simulink model "test_path_detector"  (Simulink 7.6)
settings: Solver=FixedStepDiscrete  StartTime=0.0  StopTime=0  RelTol=1e-3
undefined symbols (not defined in the file or in its folder): gray, Rec, Scale_Down_B, Scale_Down_G, Scale_Down_H, Scale_Down_R, Scale_Down_S, Scale_Down_V, SDTV
libraries: vipsnks x12, vipconversions x2, vipsrcs x1, viptextngfix x1
settings Model: Creator=Thing 1  LastModifiedBy=auvt
settings RTWCC: TargetLang=C++

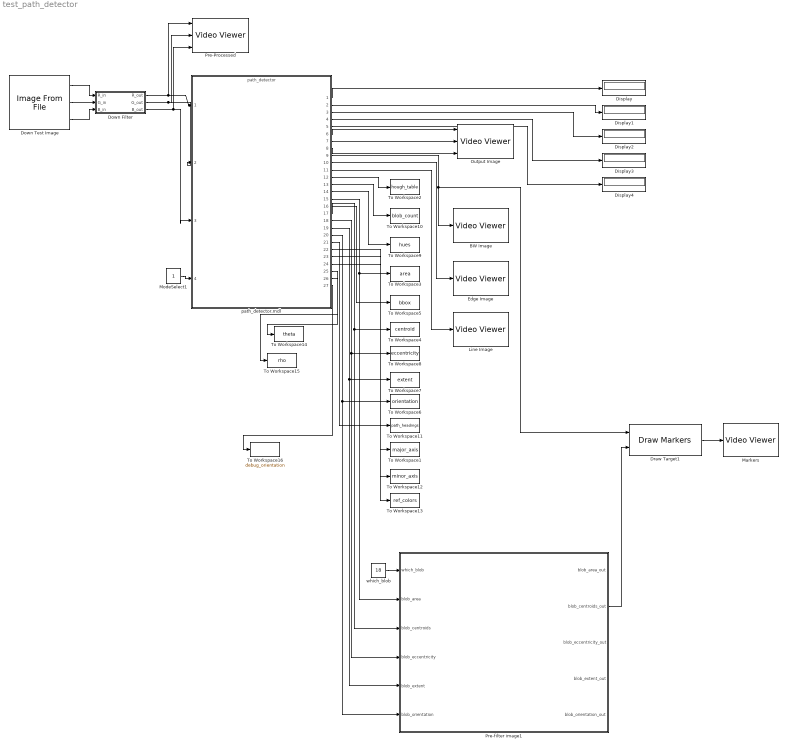
== system test_path_detector ==
  BW Image : vipsnks/Video Viewer  DialogControllerArgs=DataTag1  inputType=Obsolete7b  imagePorts=One multidimensional signal  useColorMap=off  colormapValue=gray(256)  specRange=off  minInputVal=0  maxInputVal=255  FigPos=[636 642 290 272]  AxisZoom=on  trueSizedOnce=off  OpenAtMdlStart=on
  Display{,1..4} (5 alike) : Display
  Down Filter : Subsystem
  Down Test Image : vipsrcs/Image From File  Tag=vipblks_nd  DialogController=vipDDGCreate  DialogControllerArgs=DataTag14  SystemSampleTime=-1  FileName=/home/auvt/auvc/src/vision/Test_Images/path4.PNG  imagePorts=Separate color signals  Ts=-1  ImageDataType=double  Signed=on  WordLength=16  sdImageDataType=uint(8)  FractionLengthMode=User-defined  FractionLength=15  OutPortLabels=R|G|B
  Draw Target1 : viptextngfix/Draw Markers  DialogController=vipDDGCreate  DialogControllerArgs=DataTag15  shape=X-mark  size=7  fill=off  fillClrSource=Specify via dialog  display=Black  intensity=200  color=[0 0 0]  opacity=0.6  viewport=Entire image  antialiasing=off  inType=Obsolete  imagePorts=One multidimensional signal  prodOutputMode=Binary point scaling  prodOutputWordLength=32  prodOutputFracLength=14  memoryMode=Specify word length  memoryWordLength=16  memoryFracLength=15  roundingMode=Floor  overflowMode=off
  Edge Image : vipsnks/Video Viewer  DialogControllerArgs=DataTag17  inputType=Obsolete7b  imagePorts=One multidimensional signal  useColorMap=off  colormapValue=gray(256)  specRange=off  minInputVal=0  maxInputVal=255  FigPos=[581 861 263 238]  AxisZoom=on  trueSizedOnce=off  OpenAtMdlStart=on
  Line Image : vipsnks/Video Viewer  DialogControllerArgs=DataTag19  inputType=Obsolete7b  imagePorts=One multidimensional signal  useColorMap=off  colormapValue=gray(256)  specRange=off  minInputVal=0  maxInputVal=255  FigPos=[808 631 418 354]  AxisZoom=on  trueSizedOnce=off  OpenAtMdlStart=on
  Markers : vipsnks/Video Viewer  DialogControllerArgs=DataTag21  inputType=Obsolete7b  imagePorts=One multidimensional signal  useColorMap=off  colormapValue=gray(256)  specRange=off  minInputVal=0  maxInputVal=255  FigPos=[1048 845 363 299]  AxisZoom=on  trueSizedOnce=off  OpenAtMdlStart=on
  ModeSelect1 : Constant  SampleTime=-1
  Output Image : vipsnks/Video Viewer  DialogControllerArgs=DataTag23  inputType=Obsolete7b  imagePorts=Separate color signals  useColorMap=off  colormapValue=gray(256)  specRange=off  minInputVal=0  maxInputVal=255  FigPos=[1556 512 522 277]  AxisZoom=on  trueSizedOnce=off  OpenAtMdlStart=on
  Pre-Processed : vipsnks/Video Viewer  DialogControllerArgs=DataTag25  inputType=Obsolete7b  imagePorts=Separate color signals  useColorMap=off  colormapValue=gray(256)  specRange=off  minInputVal=0  maxInputVal=255  FigPos=[2109 410 306 217]  AxisZoom=on  trueSizedOnce=off  OpenAtMdlStart=on
  Pre-filter image1 : Stateflow chart  TreatAsAtomicUnit=on
  To Workspace1 : ToWorkspace  VariableName=major_axis  SampleTime=-1  SaveFormat=Array
  To Workspace10 : ToWorkspace  VariableName=blob_count  SampleTime=-1  SaveFormat=Array
  To Workspace11 : ToWorkspace  VariableName=path_headings  SampleTime=-1  SaveFormat=Array
  To Workspace12 : ToWorkspace  VariableName=minor_axis  SampleTime=-1  SaveFormat=Array
  To Workspace13 : ToWorkspace  VariableName=ref_colors  SampleTime=-1  SaveFormat=Array
  To Workspace14 : ToWorkspace  VariableName=theta  SampleTime=-1  SaveFormat=Array
  To Workspace15 : ToWorkspace  VariableName=rho  SampleTime=-1  SaveFormat=Array
  To Workspace16 : ToWorkspace  VariableName=debug_orientation  SampleTime=-1  SaveFormat=Array
  To Workspace2 : ToWorkspace  VariableName=hough_table  SampleTime=-1  SaveFormat=Array
  To Workspace3 : ToWorkspace  VariableName=area  SampleTime=-1  SaveFormat=Array
  To Workspace4 : ToWorkspace  VariableName=centroid  SampleTime=-1  SaveFormat=Array
  To Workspace5 : ToWorkspace  VariableName=bbox  SampleTime=-1  SaveFormat=Array
  To Workspace6 : ToWorkspace  VariableName=orientation  SampleTime=-1  SaveFormat=Array
  To Workspace7 : ToWorkspace  VariableName=extent  SampleTime=-1  SaveFormat=Array
  To Workspace8 : ToWorkspace  VariableName=eccentricity  SampleTime=-1  SaveFormat=Array
  To Workspace9 : ToWorkspace  VariableName=hues  SampleTime=-1  SaveFormat=Array
  path_detector.mdl : ModelReference  ModelNameDialog=path_detector  SimulationMode=Accelerator  ModelReferenceVersion=1.185  CopyOfModelName=path_detector
  which_blob : Constant  Value=18  SampleTime=-1
  wires:
  Down Filter/1(R_out) -> path_detector.mdl/1, Pre-Processed/1
  Down Filter/2(G_out) -> path_detector.mdl/2, Pre-Processed/2
  Down Filter/3(B_out) -> path_detector.mdl/3, Pre-Processed/3
  path_detector.mdl/1 -> Display/1
  path_detector.mdl/2 -> Display1/1
  path_detector.mdl/3 -> Display2/1
  path_detector.mdl/4 -> Display3/1
  ModeSelect1/1 -> path_detector.mdl/4
  path_detector.mdl/6 -> Output Image/1
  path_detector.mdl/7 -> Output Image/2
  path_detector.mdl/8 -> Output Image/3
  path_detector.mdl/9 -> BW Image/1, Draw Target1/1
  path_detector.mdl/10 -> Edge Image/1
  path_detector.mdl/11 -> Line Image/1
  path_detector.mdl/5 -> Display4/1
  path_detector.mdl/12 -> To Workspace2/1
  path_detector.mdl/20 -> To Workspace6/1, Pre-filter image1/6(blob_orientation)
  path_detector.mdl/19 -> To Workspace7/1, Pre-filter image1/5(blob_extent)
  path_detector.mdl/18 -> To Workspace8/1, Pre-filter image1/4(blob_eccentricity)
  path_detector.mdl/17 -> To Workspace4/1, Pre-filter image1/3(blob_centroids)
  path_detector.mdl/16 -> To Workspace5/1
  path_detector.mdl/15 -> To Workspace3/1, Pre-filter image1/2(blob_area)
  path_detector.mdl/13 -> To Workspace10/1
  path_detector.mdl/14 -> To Workspace9/1
  path_detector.mdl/21 -> To Workspace11/1
  Draw Target1/1 -> Markers/1
  which_blob/1 -> Pre-filter image1/1(which_blob)
  Pre-filter image1/2(blob_centroids_out) -> Draw Target1/2
  path_detector.mdl/22 -> To Workspace1/1
  path_detector.mdl/23 -> To Workspace12/1
  path_detector.mdl/24 -> To Workspace13/1
  Down Test Image/2 -> Down Filter/2(G_in)
  Down Test Image/1 -> Down Filter/1(R_in)
  Down Test Image/3 -> Down Filter/3(B_in)
  path_detector.mdl/25 -> To Workspace14/1
  path_detector.mdl/26 -> To Workspace15/1
  path_detector.mdl/27 -> To Workspace16/1

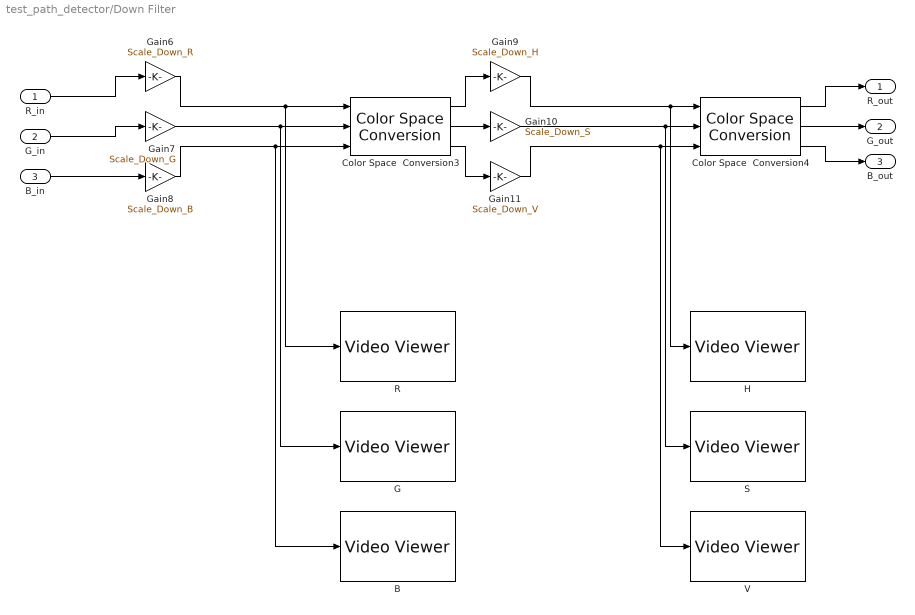
== system test_path_detector/Down Filter ==
  R_in : Inport  PortDimensions=Down_Camera_Dimensions
  G_in : Inport  Port=2  PortDimensions=Down_Camera_Dimensions
  B_in : Inport  Port=3  PortDimensions=Down_Camera_Dimensions
  B : vipsnks/Video Viewer  DialogControllerArgs=DataTag3  inputType=Obsolete7b  imagePorts=One multidimensional signal  useColorMap=off  colormapValue=gray(256)  specRange=off  minInputVal=0  maxInputVal=255  FigPos=[-198 832 410 300]  AxisZoom=on  trueSizedOnce=off  OpenAtMdlStart=on
  Color Space  Conversion3 : vipconversions/Color Space  Conversion  conversion=Obsolete  conversionActive=R'G'B' to HSV  wp_str=D50  rec=Rec. 601 (SDTV)  sys=1125/60/2:1  imagePorts=Separate color signals
  Color Space  Conversion4 : vipconversions/Color Space  Conversion  conversion=Obsolete  conversionActive=HSV to R'G'B'  wp_str=D50  rec=Rec. 601 (SDTV)  sys=1125/60/2:1  imagePorts=Separate color signals
  G : vipsnks/Video Viewer  DialogControllerArgs=DataTag5  inputType=Obsolete7b  imagePorts=One multidimensional signal  useColorMap=off  colormapValue=gray(256)  specRange=off  minInputVal=0  maxInputVal=255  FigPos=[-48 562 410 300]  AxisZoom=on  trueSizedOnce=off  OpenAtMdlStart=on
  Gain10 : Gain  Gain=Scale_Down_S
  Gain11 : Gain  Gain=Scale_Down_V
  Gain6 : Gain  Gain=Scale_Down_R
  Gain7 : Gain  Gain=Scale_Down_G
  Gain8 : Gain  Gain=Scale_Down_B
  Gain9 : Gain  Gain=Scale_Down_H
  H : vipsnks/Video Viewer  DialogControllerArgs=DataTag7  inputType=Obsolete7b  imagePorts=One multidimensional signal  useColorMap=off  colormapValue=gray(256)  specRange=off  minInputVal=0  maxInputVal=255  FigPos=[218 436 410 300]  AxisZoom=on  trueSizedOnce=off  OpenAtMdlStart=on
  R : vipsnks/Video Viewer  DialogControllerArgs=DataTag9  inputType=Obsolete7b  imagePorts=One multidimensional signal  useColorMap=off  colormapValue=gray(256)  specRange=off  minInputVal=0  maxInputVal=255  FigPos=[-120 436 410 300]  AxisZoom=on  trueSizedOnce=off  OpenAtMdlStart=on
  S : vipsnks/Video Viewer  DialogControllerArgs=DataTag11  inputType=Obsolete7b  imagePorts=One multidimensional signal  useColorMap=off  colormapValue=gray(256)  specRange=off  minInputVal=0  maxInputVal=255  FigPos=[172 632 410 300]  AxisZoom=on  trueSizedOnce=off  OpenAtMdlStart=on
  V : vipsnks/Video Viewer  DialogControllerArgs=DataTag13  inputType=Obsolete7b  imagePorts=One multidimensional signal  useColorMap=off  colormapValue=gray(256)  specRange=off  minInputVal=0  maxInputVal=255  FigPos=[196 861 410 300]  AxisZoom=on  trueSizedOnce=off  OpenAtMdlStart=on
  R_out : Outport  OutDataTypeStr=double
  G_out : Outport  Port=2  OutDataTypeStr=double
  B_out : Outport  Port=3  OutDataTypeStr=double
  wires:
  Gain6/1 -> Color Space  Conversion3/1, R/1
  Gain7/1 -> Color Space  Conversion3/2, G/1
  Gain8/1 -> Color Space  Conversion3/3, B/1
  Color Space  Conversion3/1 -> Gain9/1
  Color Space  Conversion3/2 -> Gain10/1
  Color Space  Conversion3/3 -> Gain11/1
  Gain9/1 -> Color Space  Conversion4/1, H/1
  Gain10/1 -> Color Space  Conversion4/2, S/1
  Gain11/1 -> Color Space  Conversion4/3, V/1
  R_in/1 -> Gain6/1
  G_in/1 -> Gain7/1
  B_in/1 -> Gain8/1
  Color Space  Conversion4/1 -> R_out/1
  Color Space  Conversion4/2 -> G_out/1
  Color Space  Conversion4/3 -> B_out/1

== matlab function Pre-filter image1 ==
  data: which_blob input double; blob_area input double; blob_centroids input double; blob_eccentricity input double; blob_extent input double; blob_orientation input double; blob_area_out output double; blob_centroids_out output double; blob_eccentricity_out output double; blob_extent_out output double; blob_orientation_out output double
function [blob_area_out, blob_centroids_out, blob_eccentricity_out, blob_extent_out, blob_orientation_out] = chooseBlob(which_blob, blob_area, blob_centroids, blob_eccentricity, blob_extent, blob_orientation)
%#eml

blob_area_out = blob_area(which_blob);
blob_centroids_out = blob_centroids(:,which_blob);
blob_eccentricity_out = blob_eccentricity(which_blob);
blob_extent_out = blob_extent(which_blob);
blob_orientation_out = blob_orientation(which_blob);




return
